simulink model "M1_sys_00"  (R2013b)
settings: Solver=FixedStepDiscrete  StartTime=0.0  StopTime=inf  FixedStep=0.002  MaxStep=0.002  RelTol=1e-3
values from neighbouring files (symbols this model uses):
  Cfki = 0.2*ones(1,6)    [M1DynamicModelParameters01.m]
  Cfkp = 0.0*ones(1,6)    [M1DynamicModelParameters01.m]
  CG2So = [1 0 0 0 Socg(3) -Socg(2); 0 1 0 -Socg(3) 0 Socg(1);0 0 1 Socg(2) -Socg(1) 0; 0 0 0 1 0 0; 0 0 0 0 1 0; 0 0 0 0 0 1]    [M1DynamicModelParameters01.m]
  Fscf = 100;,    [M1DynamicModelParameters01.m]
  GainM = inv(Mvect)*inv(Mm)    [M1DynamicModelParameters01.m]
  HpK = [170e6; 170e6; 170e6; 170e6; 170e6; 170e6]    [M1DynamicModelParameters01.m]
  KinematicsM = [dL_dx dL_dy dL_dz dL_drx dL_dry dL_drz]    [M1DynamicModelParameters01.m]
  KmXInvK = Km*InvKinematicsM    [M1DynamicModelParameters01.m]
  MHP = zeros(6)    [M1DynamicModelParameters01.m]
  SoKinematics = KinematicsM*inv(CG2So)    [M1DynamicModelParameters01.m]
undefined symbols (not defined in the file or in its folder): Mvect
libraries: cstblocks x12
settings Model: Creator=birarrazaval  LastModifiedBy=birarrazaval

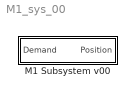
== system M1_sys_00 ==
  M1 Subsystem v00 : Subsystem  Description=|  InitFcn=M1DynamicModelParameters01  TreatAsAtomicUnit=on
      | M1 Subsystem V00
      | This subsystem models the dynamic behavior of a Primary segment as a 6 DOF rigid body.
      | The demand and position coordinates correspond to the motions  of the translations and rotations of an specific
      | Optical Surface origin.
      | This surface origin (So) is defined as the intersection of the optical surface and the axes CL in drawing 14558 page 2/6, Its global location is defined in drawing 13784  page 2/2
      | Units are in meters and radians.
      | File M1DynamicModelParameters01.m has been added in the Initfcn callback, in order to load all the constants associated to the model.
      | The dynamic behavior( Transfer Functions)  of the hard poitn motion and the mirror mass motion has been transform into discrete time format.( Z transform)
      | The Force controller is discrete in nature.
      | Simulation: Model Configuration Parameters
      | Solver type: Fixed Step
      | Solver: Discrete
      | Sample Time: 0.002 seconds

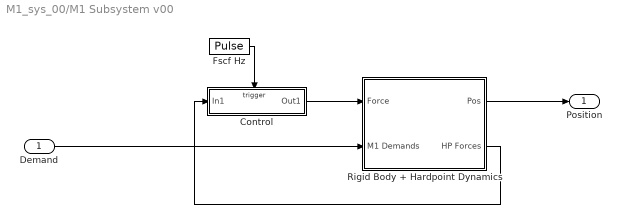
== system M1_sys_00/M1 Subsystem v00 ==
  Demand : Inport
  Control : Subsystem  TreatAsAtomicUnit=on
  Fscf Hz : DiscretePulseGenerator  Period=floor(1/(Fscf*0.002))  PhaseDelay=1  SampleTime=0.002
  Rigid Body + Hardpoint Dynamics : Subsystem  TreatAsAtomicUnit=on
  Position : Outport
  wires:
  Control/1(Out1) -> Rigid Body + Hardpoint Dynamics/1(Force)
  Fscf Hz/1 -> Control/Trigger
  Rigid Body + Hardpoint Dynamics/2(HP Forces) -> Control/1(In1)
  Rigid Body + Hardpoint Dynamics/1(Pos) -> Position/1
  Demand/1 -> Rigid Body + Hardpoint Dynamics/2(M1 Demands)

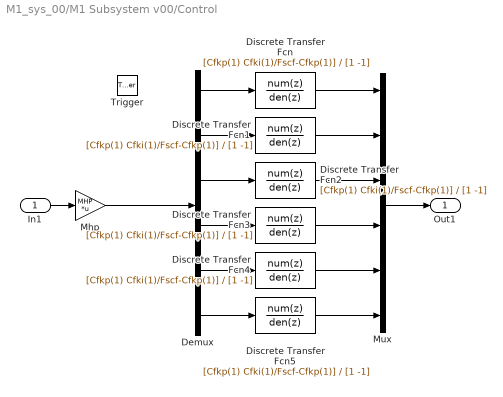
== system M1_sys_00/M1 Subsystem v00/Control ==
  In1 : Inport  LatchByDelayingOutsideSignal=on
  Trigger : TriggerPort  PortDimensions=1
  Demux : Demux  Outputs=6
  Discrete Transfer Fcn{,1..5} (6 alike) : DiscreteTransferFcn  Numerator=[Cfkp(1) Cfki(1)/Fscf-Cfkp(1)]  Denominator=[1 -1]
  Mhp : Gain  Gain=MHP  Multiplication=Matrix(K*u)
  Mux : Mux  Inputs=6
  Out1 : Outport
  wires:
  Mux/1 -> Out1/1
  Demux/1 -> Discrete Transfer Fcn/1
  Demux/2 -> Discrete Transfer Fcn1/1
  Demux/3 -> Discrete Transfer Fcn2/1
  Demux/4 -> Discrete Transfer Fcn3/1
  Demux/5 -> Discrete Transfer Fcn4/1
  Demux/6 -> Discrete Transfer Fcn5/1
  Discrete Transfer Fcn2/1 -> Mux/3
  Discrete Transfer Fcn5/1 -> Mux/6
  Discrete Transfer Fcn1/1 -> Mux/2
  Discrete Transfer Fcn4/1 -> Mux/5
  Discrete Transfer Fcn3/1 -> Mux/4
  Discrete Transfer Fcn/1 -> Mux/1
  In1/1 -> Mhp/1
  Mhp/1 -> Demux/1

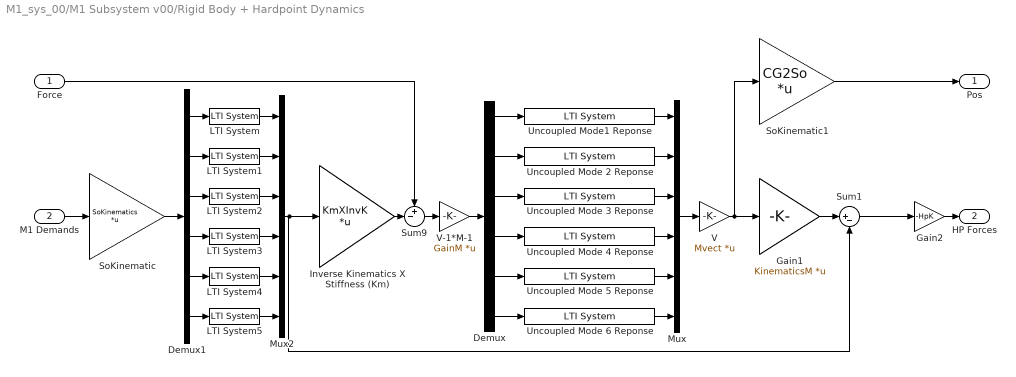
== system M1_sys_00/M1 Subsystem v00/Rigid Body + Hardpoint Dynamics ==
  Force : Inport
  M1 Demands : Inport  Port=2
  Demux : Demux  Outputs=6
  Demux1 : Demux  Outputs=6
  Gain1 : Gain  Gain=KinematicsM  Multiplication=Matrix(K*u)
  Gain2 : Gain  Gain=-HpK
  Inverse Kinematics X Stiffness (Km) : Gain  Gain=KmXInvK  Multiplication=Matrix(K*u)
  LTI System{,1..5} (6 alike) : cstblocks/LTI System  sys=HPdtf  IC=[]
  Mux : Mux  Inputs=6
  Mux2 : Mux  Inputs=6
  SoKinematic : Gain  Gain=SoKinematics  Multiplication=Matrix(K*u)
  SoKinematic1 : Gain  Gain=CG2So  Multiplication=Matrix(K*u)
  Sum1 : Sum  Inputs=|+-
  Sum9 : Sum  Inputs=+-|
  Uncoupled Mode 2 Reponse : cstblocks/LTI System  sys=Mode2MirrorTf  IC=[]
  Uncoupled Mode 3 Reponse : cstblocks/LTI System  sys=Mode3MirrorTf  IC=[]
  Uncoupled Mode 4 Reponse : cstblocks/LTI System  sys=Mode4MirrorTf  IC=[]
  Uncoupled Mode 5 Reponse : cstblocks/LTI System  sys=Mode5MirrorTf  IC=[]
  Uncoupled Mode 6 Reponse : cstblocks/LTI System  sys=Mode6MirrorTf  IC=[]
  Uncoupled Mode1 Reponse : cstblocks/LTI System  sys=Mode1MirrorTf  IC=[]
  V : Gain  Gain=Mvect  Multiplication=Matrix(K*u)
  V-1*M-1 : Gain  Gain=GainM  Multiplication=Matrix(K*u)
  Pos : Outport
  HP Forces : Outport  Port=2
  wires:
  Force/1 -> Sum9/1
  Inverse Kinematics X Stiffness (Km)/1 -> Sum9/2
  Sum9/1 -> V-1*M-1/1
  Uncoupled Mode1 Reponse/1 -> Mux/1
  Uncoupled Mode 4 Reponse/1 -> Mux/4
  Uncoupled Mode 3 Reponse/1 -> Mux/3
  Uncoupled Mode 6 Reponse/1 -> Mux/6
  Uncoupled Mode 5 Reponse/1 -> Mux/5
  Uncoupled Mode 2 Reponse/1 -> Mux/2
  Mux/1 -> V/1
  Demux/1 -> Uncoupled Mode1 Reponse/1
  Demux/2 -> Uncoupled Mode 2 Reponse/1
  Demux/3 -> Uncoupled Mode 3 Reponse/1
  Demux/4 -> Uncoupled Mode 4 Reponse/1
  Demux/5 -> Uncoupled Mode 5 Reponse/1
  Demux/6 -> Uncoupled Mode 6 Reponse/1
  V-1*M-1/1 -> Demux/1
  M1 Demands/1 -> SoKinematic/1
  LTI System1/1 -> Mux2/2
  LTI System2/1 -> Mux2/3
  LTI System3/1 -> Mux2/4
  LTI System4/1 -> Mux2/5
  LTI System5/1 -> Mux2/6
  LTI System/1 -> Mux2/1
  Demux1/1 -> LTI System/1
  Mux2/1 -> Sum1/2, Inverse Kinematics X Stiffness (Km)/1
  V/1 -> SoKinematic1/1, Gain1/1
  Demux1/2 -> LTI System1/1
  Demux1/3 -> LTI System2/1
  Demux1/4 -> LTI System3/1
  Demux1/5 -> LTI System4/1
  Demux1/6 -> LTI System5/1
  Gain2/1 -> HP Forces/1
  SoKinematic/1 -> Demux1/1
  Gain1/1 -> Sum1/1
  Sum1/1 -> Gain2/1
  SoKinematic1/1 -> Pos/1
